simulink model "BoostConvertor_Inverter_Combined"  (R2020a)
settings: Solver=VariableStepAuto  StartTime=0.0  StopTime=5  RelTol=1e-3
libraries: powerlib x24, powerlib_meascontrol x2
settings Model: Creator=alekh  LastModifiedBy=alekh

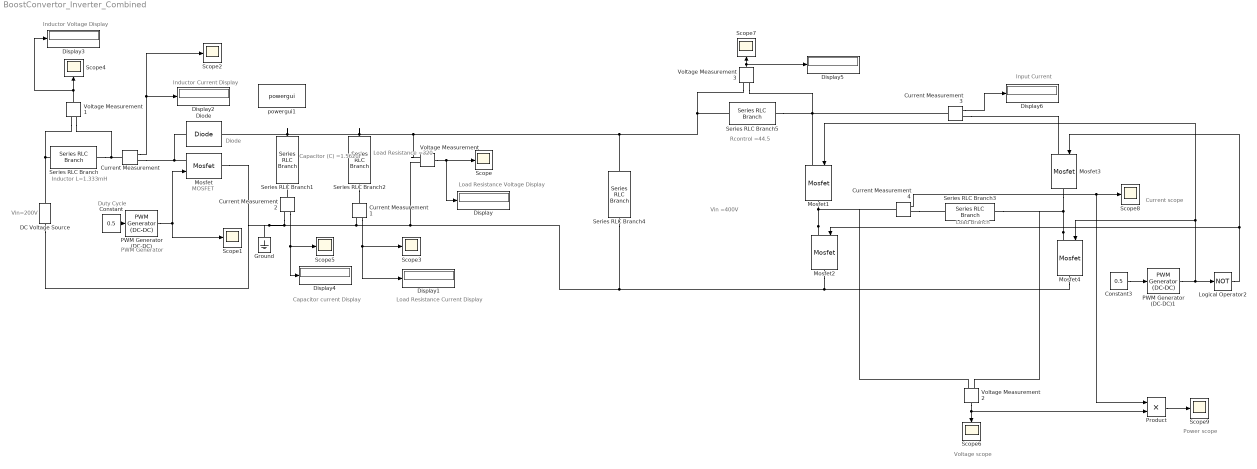
== system BoostConvertor_Inverter_Combined ==
  note: Load
      |  Resistance
      | =320
  note: Capacitor (C)
      |  =1.562uF
  note: MOSFET
  note: Diode
  note: Inductor L=1.333mH
  note: Vin=200V
  note: Duty Cycle
  note: PWM Generator
  note: Inductor Current Display
  note: Inductor Voltage Display
  note: Load Resistance Current Display
  note: Load Resistance Voltage Display
  note: Capacitor current Display
  note: Vin =400V
  note: Current scope
  note: Input Current
  note: Load Branch
  note: Power scope
  note: Rcontrol =44.5
  note: Voltage scope
  Constant : Constant  Value=0.5
  Constant3 : Constant  Value=0.5
  Current Measurement{,1..4} (5 alike) : powerlib/Measurements/Current Measurement  PhasorSimulation=off  OutputType=Complex  PSBequivalent=0
  DC Voltage Source : powerlib/Electrical Sources/DC Voltage Source  Amplitude=200  Measurements=None
  Diode : powerlib/Power Electronics/Diode  Ron=0.001  Lon=0  Vf=0.8  IC=0  UseSnubber=0  Rs=500  Cs=250e-9  Measurements=off
  Display{,1..6} (7 alike) : Display
  Ground : powerlib/Elements/Ground  LConnTagsString=a
  Logical Operator2 : Logic  Operator=NOT  AllPortsSameDT=off  OutDataTypeStr=boolean
  Mosfet{,1..4} (5 alike) : powerlib/Power Electronics/Mosfet  Ron=0.1  Lon=0  Rd=0.01  Vfd=0  IC=0  Rs=1e5  Cs=inf  Measurements=off
  PWM Generator (DC-DC) : powerlib_meascontrol/Pulse & Signal Generators/PWM Generator (DC-DC)  Fsw=100000  Ts=0
  PWM Generator (DC-DC)1 : powerlib_meascontrol/Pulse & Signal Generators/PWM Generator (DC-DC)  Fsw=50  Ts=0
  Product : Product
  Scope{,1..9} (10 alike) : Scope
  Series RLC Branch : powerlib/Elements/Series RLC Branch  LConnTagsString=__new0  RConnTagsString=__new0  BranchType=L  Resistance=1  Inductance=1.33*10^(-3)  SetiL0=off  InitialCurrent=0  Capacitance=1e-6  Setx0=off  InitialVoltage=0  Measurements=None
  Series RLC Branch1 : powerlib/Elements/Series RLC Branch  LConnTagsString=__new0  RConnTagsString=__new0  BranchType=C  Resistance=1  Inductance=1e-3  SetiL0=off  InitialCurrent=0  Capacitance=1.562*10^(-6)  Setx0=off  InitialVoltage=0  Measurements=None
  Series RLC Branch2 : powerlib/Elements/Series RLC Branch  LConnTagsString=__new0  RConnTagsString=__new0  BranchType=R  Resistance=320  Inductance=1e-3  SetiL0=off  InitialCurrent=0  Capacitance=1e-6  Setx0=off  InitialVoltage=0  Measurements=None
  Series RLC Branch3 : powerlib/Elements/Series RLC Branch  LConnTagsString=__new0  RConnTagsString=__new0  BranchType=RLC  Resistance=60  Inductance=1.5*10^(-6)  SetiL0=off  InitialCurrent=0  Capacitance=75*10^(-6)  Setx0=off  InitialVoltage=0  Measurements=None
  Series RLC Branch4 : powerlib/Elements/Series RLC Branch  LConnTagsString=__new0  RConnTagsString=__new0  BranchType=C  Resistance=1  Inductance=1e-3  SetiL0=off  InitialCurrent=0  Capacitance=1.19*10^(-3)  Setx0=off  InitialVoltage=0  Measurements=None
  Series RLC Branch5 : powerlib/Elements/Series RLC Branch  LConnTagsString=__new0  RConnTagsString=__new0  BranchType=R  Resistance=44.5  Inductance=9100*10^(-6)  SetiL0=off  InitialCurrent=0  Capacitance=1e-6  Setx0=off  InitialVoltage=0  Measurements=None
  Voltage Measurement{,1..3} (4 alike) : powerlib/Measurements/Voltage Measurement  PhasorSimulation=off  OutputType=Complex  PSBequivalent=0
  powergui1 : powerlib/powergui  Priority=1  SimulationMode=Continuous  SampleTime=5e-07  frequency=60  Iterations=50  frequencyindice=0  Pbase=100e6  ErrMax=1e-4  UnitsV=kV  UnitsW=MW  buscounter=0  FunctionMessages=off  echomessages=off  EnableUseOfTLC=off  CurrentSourceSwitches=off  DisableSnubberDevices=off  DisableRonSwitches=off  DisableVfSwitches=off  DisplayEquations=off  AutomaticDiscreteSolvers=off  SolverType=Tustin/Backward Euler (TBE)  Interpol=off  ExternalGateDelay=off  methode=off  Ts=100  x0status=blocks  SPID=on  SwTol=0  HookPort=off  NonlinearTolerance=0  nMaxIteration=15  ContinueOnMaxIteration=off  RestoreLinks=warning  ResistiveCurrentMeasurement=off  Frange=[0:2:500]  Ylog=off  Xlog=on  ShowGrid=off  save=off  variable=ZData  structure=0  ZoomFFT=off  StartTime=0.0  cycles=1  DisplayStyle=1  fundamental=60  FreqAxis=off  MaxFrequency=1000  frequencyindicesteady=1  RmsSteady=1  display=off
  wires:
  PWM Generator (DC-DC)/1 -> Mosfet/1, Scope1/1
  Constant/1 -> PWM Generator (DC-DC)/1
  Voltage Measurement/1 -> Scope/1, Display/1
  Current Measurement/1 -> Display2/1, Scope2/1
  Current Measurement1/1 -> Display1/1, Scope3/1
  Voltage Measurement1/1 -> Display3/1, Scope4/1
  Current Measurement2/1 -> Display4/1, Scope5/1
  Product/1 -> Scope9/1
  Constant3/1 -> PWM Generator (DC-DC)1/1
  Current Measurement4/1 -> Product/1, Scope8/1
  Current Measurement3/1 -> Display6/1
  PWM Generator (DC-DC)1/1 -> Logical Operator2/1, Mosfet1/1, Mosfet4/1
  Voltage Measurement3/1 -> Display5/1, Scope7/1
  Logical Operator2/1 -> Mosfet3/1, Mosfet2/1
  Voltage Measurement2/1 -> Scope6/1, Product/2
  connections:
  Diode/LConn1 -- Mosfet/LConn1 -- Current Measurement/RConn1
  Voltage Measurement3/LConn1 -- Series RLC Branch4/LConn1 -- Series RLC Branch1/LConn1 -- Diode/RConn1 -- Series RLC Branch2/LConn1 -- Voltage Measurement/LConn1 -- Series RLC Branch5/LConn1
  Mosfet4/RConn1 -- Mosfet2/RConn1 -- Series RLC Branch4/RConn1 -- Mosfet/RConn1 -- DC Voltage Source/LConn1 -- Ground/LConn1 -- Current Measurement2/RConn1 -- Current Measurement1/RConn1 -- Voltage Measurement/LConn2
  DC Voltage Source/RConn1 -- Series RLC Branch/LConn1 -- Voltage Measurement1/LConn1
  Series RLC Branch/RConn1 -- Voltage Measurement1/LConn2 -- Current Measurement/LConn1
  Series RLC Branch2/RConn1 -- Current Measurement1/LConn1
  Current Measurement2/LConn1 -- Series RLC Branch1/RConn1
  Mosfet4/LConn1 -- Mosfet3/RConn1 -- Voltage Measurement2/LConn2 -- Series RLC Branch3/RConn1
  Mosfet2/LConn1 -- Mosfet1/RConn1 -- Voltage Measurement2/LConn1 -- Current Measurement4/LConn1
  Series RLC Branch5/RConn1 -- Current Measurement3/LConn1 -- Voltage Measurement3/LConn2 -- Mosfet1/LConn1
  Current Measurement3/RConn1 -- Mosfet3/LConn1
  Current Measurement4/RConn1 -- Series RLC Branch3/LConn1
